simulink model "lab5"  (R2022b)
settings: Solver=FixedStepAuto  StartTime=0.0  StopTime=50  FixedStep=0.001  RelTol=1e-3
undefined symbols (not defined in the file): c, k, m
settings Model: Creator=dambi  LastModifiedBy=dambi

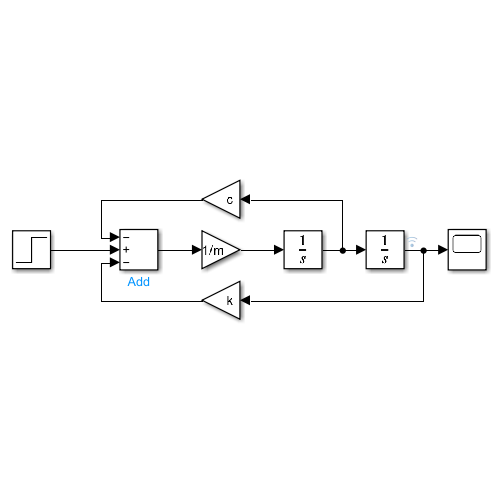
[thumbnail: Simulink's stored preview of the top-level diagram]
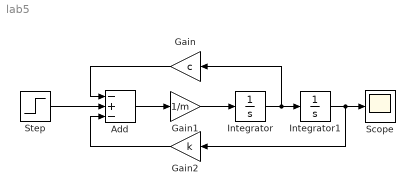
== system lab5 ==
  Add : Sum  Inputs=-+-
  Gain : Gain  Gain=c
  Gain1 : Gain  Gain=1/m
  Gain2 : Gain  Gain=k
  Integrator : Integrator
  Integrator1 : Integrator
  Scope : Scope
  Step : Step  SampleTime=0
  wires:
  Step/1 -> Add/2
  Add/1 -> Gain1/1
  Integrator/1 -> Gain/1, Integrator1/1
  Gain1/1 -> Integrator/1
  Integrator1/1 -> Gain2/1, Scope/1
  Gain2/1 -> Add/3
  Gain/1 -> Add/1
